simulink model "tanquesSimulink"  (R2018a)
settings: Solver=ode45  StartTime=0.0  StopTime=1000  RelTol=1e-6
values from neighbouring files (symbols this model uses):
  A1 = 1    [main.m]    (also in tankmodel.m = par.A1)
  a1s = 0.5    [main.m]
  A2 = 1.5    [main.m]    (also in tankmodel.m = par.A2)
  a2s = 0.45    [main.m]
  du = 0.001    [main.m]
  h1s = X(1)    [main.m]
  h2s = X(2)    [main.m]
  k1 = 0.04    [main.m]    (also in tankmodel.m = par.k1)
  k2 = 0.03    [main.m]    (also in tankmodel.m = par.k2)
  k3 = 0.055    [main.m]    (also in tankmodel.m = par.k3)
undefined symbols (not defined in the file or in its folder): par
libraries: cstblocks x1
settings Model: Creator=Sergio  LastModifiedBy=Sergio
settings CodeAppCC: StateflowObjectComments=on

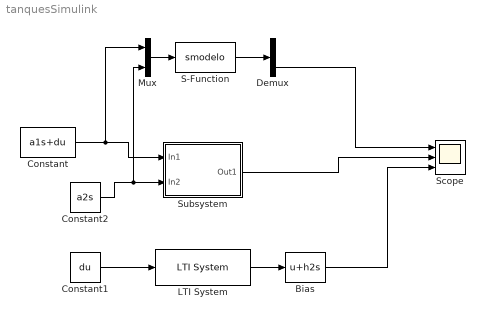
== system tanquesSimulink ==
  Bias : Bias  Bias=h2s
  Constant : Constant  Value=a1s+du
  Constant1 : Constant  Value=du
  Constant2 : Constant  Value=a2s
  Demux : Demux  Outputs=2
  LTI System : cstblocks/LTI System  sys=G  IC=[]
  Mux : Mux  Inputs=2
  S-Function : S-Function  FunctionName=smodelo  Parameters=par,h1s,h2s  SFunctionDeploymentMode=off  EnableBusSupport=off
  Scope : Scope  NumInputPorts=3
  Subsystem : Subsystem
  wires:
  Constant/1 -> Mux/1, Subsystem/1(In1)
  Constant2/1 -> Mux/2, Subsystem/2(In2)
  Mux/1 -> S-Function/1
  S-Function/1 -> Demux/1
  LTI System/1 -> Bias/1
  Constant1/1 -> LTI System/1
  Demux/2 -> Scope/1
  Subsystem/1(Out1) -> Scope/2
  Bias/1 -> Scope/3

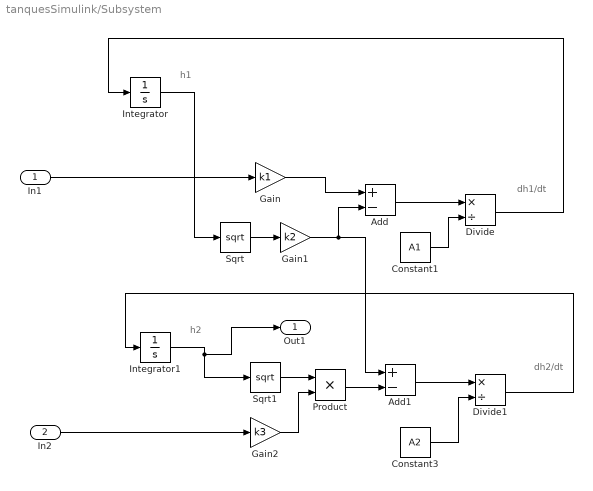
== system tanquesSimulink/Subsystem ==
  note: dh1/dt
  note: h1
  note: dh2/dt
  note: h2
  In1 : Inport
  In2 : Inport  Port=2
  Add : Sum  Inputs=+-
  Add1 : Sum  Inputs=+-
  Constant1 : Constant  Value=A1
  Constant3 : Constant  Value=A2
  Divide : Product  Inputs=*/
  Divide1 : Product  Inputs=*/
  Gain : Gain  Gain=k1
  Gain1 : Gain  Gain=k2
  Gain2 : Gain  Gain=k3
  Integrator : Integrator  InitialCondition=h1s
  Integrator1 : Integrator  InitialCondition=h2s
  Product : Product
  Sqrt : Sqrt  SaturateOnIntegerOverflow=on
  Sqrt1 : Sqrt  SaturateOnIntegerOverflow=on
  Out1 : Outport
  wires:
  Integrator/1 -> Sqrt/1
  In1/1 -> Gain/1
  Gain2/1 -> Product/2
  Add/1 -> Divide/1
  Product/1 -> Add1/2
  Gain1/1 -> Add1/1, Add/2
  Divide/1 -> Integrator/1
  Constant1/1 -> Divide/2
  Gain/1 -> Add/1
  Sqrt/1 -> Gain1/1
  Add1/1 -> Divide1/1
  Sqrt1/1 -> Product/1
  Constant3/1 -> Divide1/2
  In2/1 -> Gain2/1
  Divide1/1 -> Integrator1/1
  Integrator1/1 -> Out1/1, Sqrt1/1
